simulink model "L19Pendsim"  (R2020a)
settings: Solver=FixedStepAuto  StartTime=0.0  StopTime=100  FixedStep=0.01  RelTol=1e-3
InitFcn:
  | L19ParametersPend;
values from neighbouring files (symbols this model uses):
  A = [0 1 ; g/l -r/(m*l^2)]    [L19ParametersPend.m]
  B = [0 ; 1/(m*l^2)]    [L19ParametersPend.m]
  C = [1 0]    [L19ParametersPend.m]
  L = place(A',C',[-15 -20])'    [L19ParametersPend.m]
  x0 = [theta0 ; thetadot0]    [L19ParametersPend.m]
  x0hat = [x0(1); 0]    [L19ParametersPend.m]
settings Model: Creator=vcichella  LastModifiedBy=vcichella

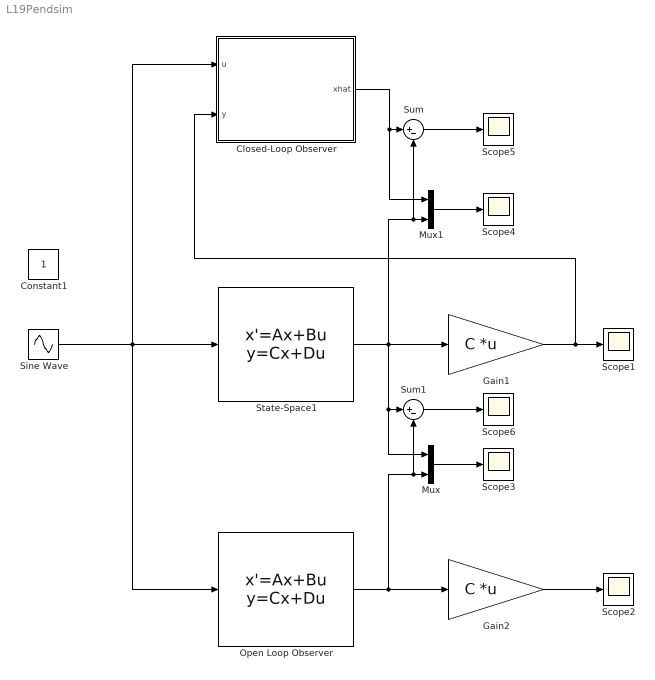
== system L19Pendsim ==
  Closed-Loop Observer : Subsystem
  Constant1 : Constant
  Gain1 : Gain  Gain=C  Multiplication=Matrix(K*u)
  Gain2 : Gain  Gain=C  Multiplication=Matrix(K*u)
  Mux : Mux  Inputs=2
  Mux1 : Mux  Inputs=2
  Open Loop Observer : StateSpace  A=A  B=B  C=eye(size(A))  D=zeros(2,1)  InitialCondition=[x0(1) 0]'
  Scope{1..6} (6 alike) : Scope
  Sine Wave : Sin  Frequency=0.1  SampleTime=0
  State-Space1 : StateSpace  A=A  B=B  C=eye(size(A))  D=zeros(2,1)  InitialCondition=x0
  Sum : Sum  Inputs=|+-
  Sum1 : Sum  Inputs=|+-
  wires:
  Gain1/1 -> Closed-Loop Observer/2(y), Scope1/1
  State-Space1/1 -> Sum/2, Mux1/2, Sum1/1, Mux/1, Gain1/1
  Sine Wave/1 -> Open Loop Observer/1, Closed-Loop Observer/1(u), State-Space1/1
  Open Loop Observer/1 -> Sum1/2, Mux/2, Gain2/1
  Gain2/1 -> Scope2/1
  Mux/1 -> Scope3/1
  Mux1/1 -> Scope4/1
  Closed-Loop Observer/1(xhat) -> Sum/1, Mux1/1
  Sum/1 -> Scope5/1
  Sum1/1 -> Scope6/1

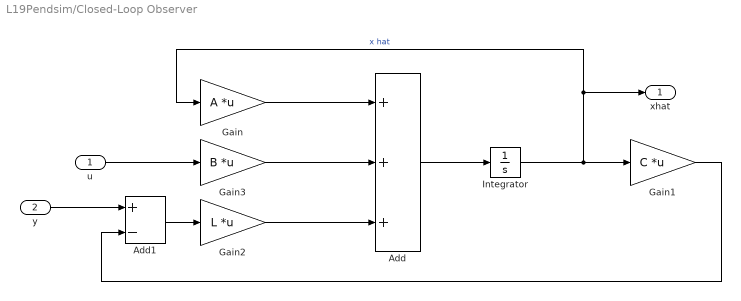
== system L19Pendsim/Closed-Loop Observer ==
  u : Inport
  y : Inport  Port=2
  Add : Sum  Inputs=+++
  Add1 : Sum  Inputs=+-
  Gain : Gain  Gain=A  Multiplication=Matrix(K*u)
  Gain1 : Gain  Gain=C  Multiplication=Matrix(K*u)
  Gain2 : Gain  Gain=L  Multiplication=Matrix(K*u)
  Gain3 : Gain  Gain=B  Multiplication=Matrix(K*u)
  Integrator : Integrator  InitialCondition=x0hat
  xhat : Outport
  wires:
  Integrator/1 -> Gain/1, xhat/1, Gain1/1  "x hat"
  Add/1 -> Integrator/1
  Gain/1 -> Add/1
  Gain1/1 -> Add1/2
  Add1/1 -> Gain2/1
  y/1 -> Add1/1
  Gain2/1 -> Add/3
  u/1 -> Gain3/1
  Gain3/1 -> Add/2
